simulink model "RailP_VD"  (R2016b)
settings: configuration reference "CodeGenConfigSet" (kept outside this file)
values from neighbouring files (symbols this model uses):
  RailP_facFlt1PT1_C = Calibration.Parameter    [init_RailP_VD.m]
  RailP_facFlt2PT1_C = Calibration.Parameter    [init_RailP_VD.m]
  RailP_facFlt3PT1_C = Calibration.Parameter    [init_RailP_VD.m]
  RailP_nDiffMax_C = Calibration.Parameter    [init_RailP_VD.m]
  RailP_numMax_CUR = Calibration.Parameter    [init_RailP_VD.m]
  RailP_numMax_CURX = Calibration.Parameter    [init_RailP_VD.m]
  RailP_pFltWinNeg_CUR = Calibration.Parameter    [init_RailP_VD.m]
  RailP_pFltWinNeg_CURX = Calibration.Parameter    [init_RailP_VD.m]
  RailP_pSubsCtlDlvMeUn_CUR = Calibration.Parameter    [init_RailP_VD.m]
  RailP_pSubsCtlDlvMeUn_CURX = Calibration.Parameter    [init_RailP_VD.m]
  RailP_swtFlt_C = Calibration.Parameter    [init_RailP_VD.m]
undefined symbols (not defined in the file or in its folder): RailCtl_State_conv
libraries: CXLib x1
settings Model: Creator=Administrator  LastModifiedBy=liutao
settings ConfigSetRef: SourceLocation=Base Workspace

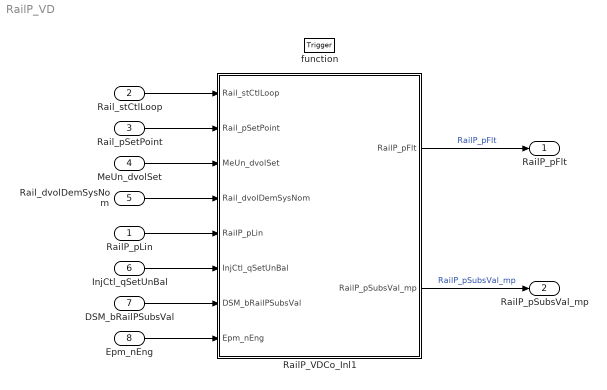
== system RailP_VD ==
  RailP_pLin : Inport  Tag=bar  Description=Fuel pressure  OutMin=0  OutMax=2500  OutDataTypeStr=RailPressure_bar
  Rail_stCtlLoop : Inport  Description=State of the rail pressure governor control  Port=2  OutDataTypeStr=Enum: RailCtl_State_conv
  Rail_pSetPoint : Inport  Tag=bar  Description=Rail pressure setpoint  Port=3  OutMin=-2500  OutMax=2500  OutDataTypeStr=RailPressure_bar
  MeUn_dvolSet : Inport  Tag=mm^3/s  Description=Setpoint value (volume flow) of rail pressure governing  Port=4  OutMin=-327670  OutMax=327670  OutDataTypeStr=FuelVol_mm3_s
  Rail_dvolDemSysNom : Inport  Tag=mm^3/s  Description=Volume flow demanded overall for a nominal injection system  Port=5  OutMin=-327680  OutMax=327670  OutDataTypeStr=FuelVol_mm3_s
  InjCtl_qSetUnBal : Inport  Tag=mg/hub  Description=Current injection quantity  Port=6  OutMin=-319  OutMax=319  OutDataTypeStr=FuelMass_mg_hub
  DSM_bRailPSubsVal : Inport  Description=Status of FId_RailPSubsVal  Port=7  OutMin=0  OutMax=1  OutDataTypeStr=boolean
  Epm_nEng : Inport  Tag=rpm  Description=Engine speed  Port=8  OutMin=0  OutMax=6000  OutDataTypeStr=EngSpeed_rpm
  function : TriggerPort  TriggerType=function-call  VariantControl=Variant
  RailP_VDCo_Inl1 : Subsystem
  RailP_pFlt : Outport  Tag=bar  Description=Maximum rail pressure of the last 10 sampling cycle  OutMin=0  OutMax=2500  OutDataTypeStr=RailPressure_bar
  RailP_pSubsVal_mp : Outport  Tag=bar  Description=Rail pressure substitution value in case of an error in pressure sensor  Port=2  OutMin=0  OutMax=2500  OutDataTypeStr=RailPressure_bar
  wires:
  Rail_pSetPoint/1 -> RailP_VDCo_Inl1/2(Rail_pSetPoint)
  Rail_stCtlLoop/1 -> RailP_VDCo_Inl1/1(Rail_stCtlLoop)
  Rail_dvolDemSysNom/1 -> RailP_VDCo_Inl1/4(Rail_dvolDemSysNom)
  MeUn_dvolSet/1 -> RailP_VDCo_Inl1/3(MeUn_dvolSet)
  RailP_VDCo_Inl1/1(RailP_pFlt) -> RailP_pFlt/1  "RailP_pFlt"
  DSM_bRailPSubsVal/1 -> RailP_VDCo_Inl1/7(DSM_bRailPSubsVal)
  InjCtl_qSetUnBal/1 -> RailP_VDCo_Inl1/6(InjCtl_qSetUnBal)
  RailP_pLin/1 -> RailP_VDCo_Inl1/5(RailP_pLin)
  Epm_nEng/1 -> RailP_VDCo_Inl1/8(Epm_nEng)
  RailP_VDCo_Inl1/2(RailP_pSubsVal_mp) -> RailP_pSubsVal_mp/1  "RailP_pSubsVal_mp"

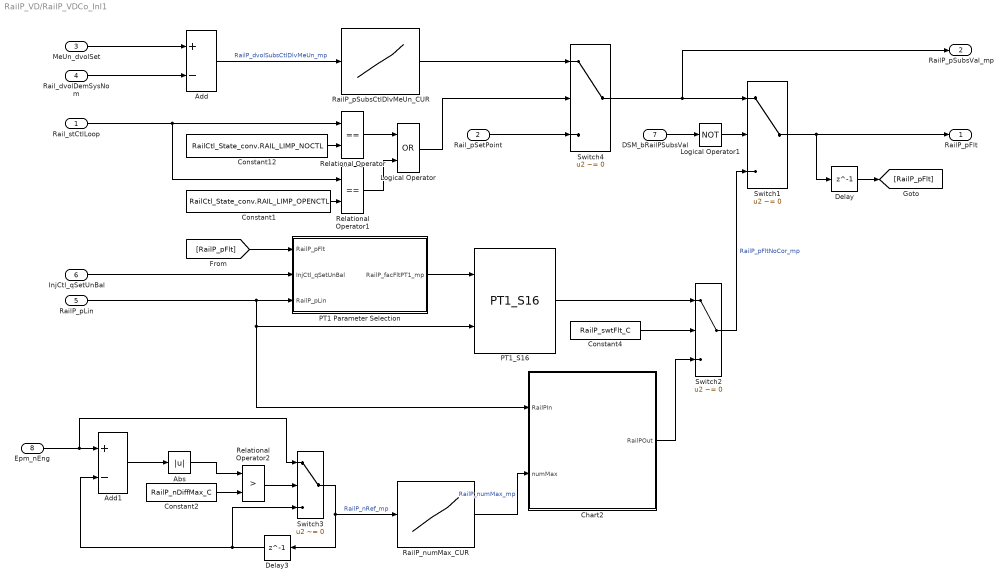
== system RailP_VD/RailP_VDCo_Inl1 ==
  Rail_stCtlLoop : Inport
  Rail_pSetPoint : Inport  Port=2
  MeUn_dvolSet : Inport  Port=3
  Rail_dvolDemSysNom : Inport  Port=4
  RailP_pLin : Inport  Tag=bar  Description=Fuel pressure  Port=5  OutMin=0  OutMax=2500  OutDataTypeStr=RailPressure_bar
  InjCtl_qSetUnBal : Inport  Tag=mg/hub  Description=current injection quantity  Port=6  OutMin=-300  OutMax=300  OutDataTypeStr=FuelMass_mg_hub
  DSM_bRailPSubsVal : Inport  Description=Status of FId_RailPSubsVal  Port=7  OutMin=0  OutMax=1  OutDataTypeStr=boolean
  Epm_nEng : Inport  Port=8
  Abs : Abs
  Add : Sum  Inputs=+-  OutDataTypeStr=Inherit: Inherit via back propagation  InputSameDT=on
  Add1 : Sum  Inputs=+-  OutDataTypeStr=Inherit: Inherit via back propagation  RndMeth=Round  InputSameDT=on
  Chart2 : Stateflow chart  TreatAsAtomicUnit=on
  Constant1 : Constant  Value=RailCtl_State_conv.RAIL_LIMP_OPENCTL  OutDataTypeStr=Inherit: Inherit via back propagation
  Constant12 : Constant  Value=RailCtl_State_conv.RAIL_LIMP_NOCTL  OutDataTypeStr=Inherit: Inherit via back propagation
  Constant2 : Constant  Value=RailP_nDiffMax_C
  Constant4 : Constant  Value=RailP_swtFlt_C
  Delay : Delay  DelayLength=1  InitialCondition=0
  Delay3 : Delay  DelayLength=1  InitialCondition=0
  Logical Operator : Logic  Operator=OR  OutDataTypeStr=boolean
  Logical Operator1 : Logic  Operator=NOT  AllPortsSameDT=off  OutDataTypeStr=boolean
  PT1 Parameter Selection : Subsystem
  PT1_S16 : CXLib/PT1_S16
  RailP_numMax_CUR : Lookup_n-D  NumberOfTableDimensions=1  BreakpointsForDimension1=RailP_numMax_CURX  IndexSearchMethod=Linear search  BeginIndexSearchUsingPreviousIndexResult=on  UseOneInputPortForAllInputData=on  Table=RailP_numMax_CUR  ExtrapMethod=Clip  UseLastTableValue=on  InternalRulePriority=Speed  OutDataTypeStr=Inherit: Inherit via back propagation  SaturateOnIntegerOverflow=on
  RailP_pSubsCtlDlvMeUn_CUR : Lookup_n-D  NumberOfTableDimensions=1  BreakpointsForDimension1=RailP_pSubsCtlDlvMeUn_CURX  IndexSearchMethod=Linear search  BeginIndexSearchUsingPreviousIndexResult=on  UseOneInputPortForAllInputData=on  Table=RailP_pSubsCtlDlvMeUn_CUR  ExtrapMethod=Clip  UseLastTableValue=on  InternalRulePriority=Speed  OutDataTypeStr=Inherit: Inherit via back propagation  SaturateOnIntegerOverflow=on
  Relational Operator : RelationalOperator  Operator===  OutDataTypeStr=boolean  RndMeth=Nearest  InputSameDT=on
  Relational Operator1 : RelationalOperator  Operator===  OutDataTypeStr=boolean  RndMeth=Nearest  InputSameDT=on
  Relational Operator2 : RelationalOperator  Operator=>  OutDataTypeStr=boolean  RndMeth=Nearest  InputSameDT=on
  Switch{1..4} (4 alike) : Switch  Criteria=u2 ~= 0  InputSameDT=on
  RailP_pFlt : Outport  Description=Maximum rail pressure of the last 10 sampling cycle
  RailP_pSubsVal_mp : Outport  Description=Maximum rail pressure of the last 10 sampling cycle  Port=2
  wires:
  Logical Operator1/1 -> Switch1/2
  Switch1/1 -> RailP_pFlt/1, Delay/1
  Switch4/1 -> RailP_pSubsVal_mp/1, Switch1/1
  DSM_bRailPSubsVal/1 -> Logical Operator1/1
  Add/1 -> RailP_pSubsCtlDlvMeUn_CUR/1  "RailP_dvolSubsCtlDlvMeUn_mp"
  RailP_pSubsCtlDlvMeUn_CUR/1 -> Switch4/1
  Constant1/1 -> Relational Operator1/2
  Logical Operator/1 -> Switch4/2
  Relational Operator1/1 -> Logical Operator/2
  Relational Operator/1 -> Logical Operator/1
  Constant12/1 -> Relational Operator/2
  PT1 Parameter Selection/1(RailP_facFltPT1_mp) -> PT1_S16/1
  Switch2/1 -> Switch1/3  "RailP_pFltNoCor_mp"
  InjCtl_qSetUnBal/1 -> PT1 Parameter Selection/2(InjCtl_qSetUnBal)
  RailP_pLin/1 -> PT1 Parameter Selection/3(RailP_pLin), Chart2/1(RailPIn), PT1_S16/2
  MeUn_dvolSet/1 -> Add/1
  Rail_dvolDemSysNom/1 -> Add/2
  Rail_stCtlLoop/1 -> Relational Operator1/1, Relational Operator/1
  Rail_pSetPoint/1 -> Switch4/3
  Constant4/1 -> Switch2/2
  PT1_S16/1 -> Switch2/1
  Epm_nEng/1 -> Switch3/1, Add1/1
  Add1/1 -> Abs/1
  Abs/1 -> Relational Operator2/1
  Constant2/1 -> Relational Operator2/2
  Relational Operator2/1 -> Switch3/2
  Switch3/1 -> Delay3/1, RailP_numMax_CUR/1  "RailP_nRef_mp"
  RailP_numMax_CUR/1 -> Chart2/2(numMax)  "RailP_numMax_mp"
  Delay3/1 -> Add1/2, Switch3/3
  Chart2/1(RailPOut) -> Switch2/3
  Delay/1 -> [RailP_pFlt]
  [RailP_pFlt] -> PT1 Parameter Selection/1(RailP_pFlt)

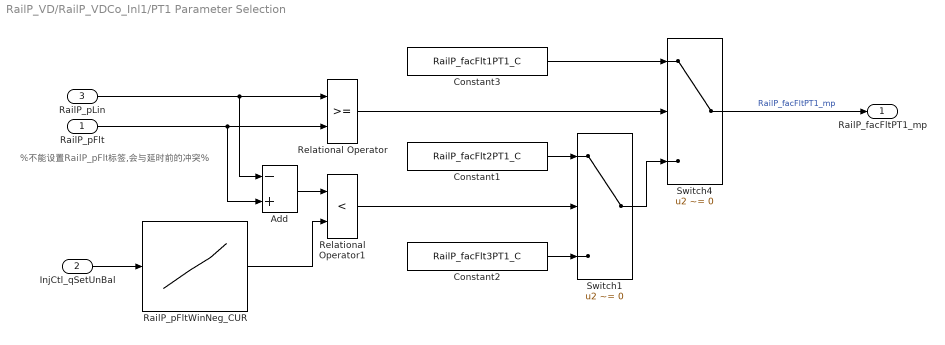
== system RailP_VD/RailP_VDCo_Inl1/PT1 Parameter Selection ==
  note: %不能设置RailP_pFlt标签,会与延时前的冲突%
  RailP_pFlt : Inport  Tag=mg/hub  Description=current injection quantity  OutMin=-300  OutMax=300
  InjCtl_qSetUnBal : Inport  Tag=mg/hub  Description=current injection quantity  Port=2  OutMin=-300  OutMax=300  OutDataTypeStr=FuelMass_mg_hub
  RailP_pLin : Inport  Tag=bar  Description=Fuel pressure  Port=3  OutMin=0  OutMax=2500  OutDataTypeStr=RailPressure_bar
  Add : Sum  Inputs=-+  OutDataTypeStr=Inherit: Inherit via back propagation  InputSameDT=on
  Constant1 : Constant  Value=RailP_facFlt2PT1_C
  Constant2 : Constant  Value=RailP_facFlt3PT1_C
  Constant3 : Constant  Value=RailP_facFlt1PT1_C
  RailP_pFltWinNeg_CUR : Lookup_n-D  NumberOfTableDimensions=1  BreakpointsForDimension1=RailP_pFltWinNeg_CURX  IndexSearchMethod=Linear search  BeginIndexSearchUsingPreviousIndexResult=on  UseOneInputPortForAllInputData=on  Table=RailP_pFltWinNeg_CUR  ExtrapMethod=Clip  UseLastTableValue=on  InternalRulePriority=Speed  OutDataTypeStr=Inherit: Inherit via back propagation  SaturateOnIntegerOverflow=on
  Relational Operator : RelationalOperator  OutDataTypeStr=boolean  RndMeth=Nearest  InputSameDT=on
  Relational Operator1 : RelationalOperator  Operator=<  OutDataTypeStr=boolean  RndMeth=Nearest  InputSameDT=on
  Switch1 : Switch  Criteria=u2 ~= 0  InputSameDT=on
  Switch4 : Switch  Criteria=u2 ~= 0  InputSameDT=on
  RailP_facFltPT1_mp : Outport
  wires:
  Constant2/1 -> Switch1/3
  Constant1/1 -> Switch1/1
  InjCtl_qSetUnBal/1 -> RailP_pFltWinNeg_CUR/1
  RailP_pFltWinNeg_CUR/1 -> Relational Operator1/2
  Add/1 -> Relational Operator1/1
  Relational Operator1/1 -> Switch1/2
  Switch1/1 -> Switch4/3
  Switch4/1 -> RailP_facFltPT1_mp/1  "RailP_facFltPT1_mp"
  Constant3/1 -> Switch4/1
  Relational Operator/1 -> Switch4/2
  RailP_pFlt/1 -> Relational Operator/2, Add/2
  RailP_pLin/1 -> Relational Operator/1, Add/1

== stateflow chart RailP_VD/RailP_VDCo_Inl1/Chart2 ==
  (default) -> (junction 2) : {i=9;}
  (junction 2) -> (junction 5) [order 1] : [i>=1]
  (junction 5) -> (junction 7) : {RailPArray[i]=RailPArray[i-1];}
  (junction 7) -> (junction 2) : {i--;}
  (junction 2) -> (junction 1) [order 2] : {i=0;
      | RailPArray[0]=RailPIn;
      | RailPMax=RailPArray[0];}
  (junction 10) -> (junction 12) [order 1] : [RailPMax<RailPArray[i]]
  (junction 1) -> (junction 10) [order 1] : [i<numMax]
  (junction 10) -> (junction 16) [order 2]
  (junction 12) -> (junction 14) : {RailPMax=RailPArray[i];}
  (junction 16) -> (junction 1) : {i++;}
  (junction 1) -> (junction 20) [order 2] : {RailPOut=RailPMax;}
  (junction 14) -> (junction 16)
  data: RailPIn input; numMax input; RailPOut output; i local uint8; RailPMax local RailPressure_bar; RailPArray local RailPressure_bar size=10
